simulink model "CoreXY_model_PWM_X"  (R2024b)
settings: Solver=VariableStepAuto  StartTime=0.0  StopTime=max(data.Time_ms_)/1000  RelTol=1e-3
values from neighbouring files (symbols this model uses):
  Kff = 2/PULLEY_RADIUS*(x1*s^3+x2*s^2+x3*s)    [CoreXY_analysis_func.m]    (also in feedforward_tuning.m)
undefined symbols (not defined in the file or in its folder): A, B, C, D, data, L, theta_to_xy, xy_cm_to_theta_rad
libraries: slpidlib x2
settings Model: Creator=trent  LastModifiedBy=mauro
settings OptimizationCC: ReuseModelBlockBuffer=off
settings DebuggingCC: UnconnectedInputMsg=warning  UnconnectedOutputMsg=warning  UnconnectedLineMsg=warning
settings ModelReferenceCC: EnableRefExpFcnMdlSchedulingChecks=on
settings RTWCC: GPUComputeCapability=3.5  DLArmComputeVersion=19.05

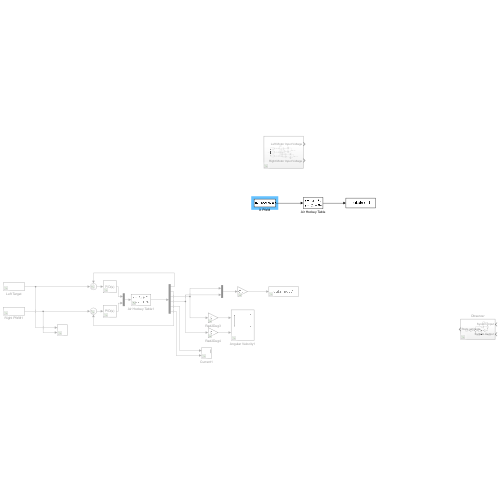
[thumbnail: Simulink's stored preview of the top-level diagram]
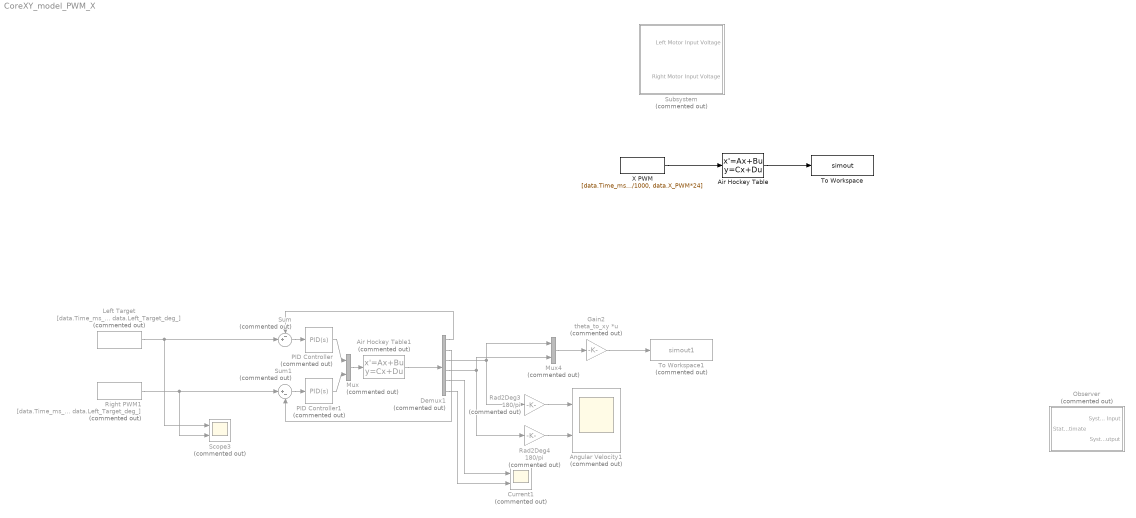
== system CoreXY_model_PWM_X ==
  Air Hockey Table : StateSpace  A=A  B=B  C=C  D=D  InitialCondition=[data.X_Accel_m_s2_(1)/C(1,3);data.X_Velocity_m_s_(1)/C(1,3);data.x(1)/C(1,3)]
  Air Hockey Table1 : StateSpace  Commented=on  A=A  B=B  C=[C; zeros(4,2) eye(4)]  D=[D; zeros(4,2)]  InitialCondition=[0;0;0;0;0;0];
  Angular Velocity1 : Scope  Commented=on  NumInputPorts=2
  Current1 : Scope  Commented=on  NumInputPorts=2
  Demux1 : Demux  Commented=on  Outputs=6
  Gain2 : Gain  Commented=on  Gain=theta_to_xy  Multiplication=Matrix(K*u)
  Left Target : FromWorkspace  Commented=on  VariableName=[data.Time_ms_/1000, data.Left_Target_deg_]
  Mux : Mux  Commented=on  Inputs=2
  Mux4 : Mux  Commented=on  Inputs=2
  Observer : Subsystem  Commented=on
  PID Controller : slpidlib/PID Controller  Commented=on  Controller=PID  Form=Parallel  TimeDomain=Continuous-time  UseExternalTs=off  SampleTime=-1  IntegratorMethod=Forward Euler  FilterMethod=Forward Euler  ControllerParametersSource=internal  P=1  I=1  UseKiTs=off  D=0  UseExternalDerivativeSource=off  N=100  UseFilter=on  TunerSelectOption=Transfer Function Based (PID Tuner App)  InitialConditionSource=internal  InitialConditionForIntegrator=0  InitialConditionForFilter=0  DifferentiatorICPrevScaledInput=0  ExternalReset=none  TrackingMode=off  Kt=1  LimitOutput=off  SatLimitsSource=internal  UpperSaturationLimit=inf  LowerSaturationLimit=-inf  LinearizeAsGain=on  AntiWindupMode=none  Kb=1  LimitIntegrator=off  UpperIntegratorSaturationLimit=inf  LowerIntegratorSaturationLimit=-inf  POutMin=[]  POutMax=[]  IOutMin=[]  IOutMax=[]  DOutMin=[]  DOutMax=[]  NOutMin=[]  NOutMax=[]  SumOutMin=[]  SumOutMax=[]  SaturationOutMin=[]  SaturationOutMax=[]  PParamMin=[]  PParamMax=[]  IParamMin=[]  IParamMax=[]  DParamMin=[]  DParamMax=[]  NParamMin=[]  NParamMax=[]  KbParamMin=[]  KbParamMax=[]  KtParamMin=[]  KtParamMax=[]  KbOutMin=[]  KbOutMax=[]  KtOutMin=[]  KtOutMax=[]  IntegratorOutMin=[]  IntegratorOutMax=[]  FilterOutMin=[]  FilterOutMax=[]  SumI1OutMin=[]  SumI1OutMax=[]  SumI2OutMin=[]  SumI2OutMax=[]  SumI3OutMin=[]  SumI3OutMax=[]  SumI4OutMin=[]  SumI4OutMax=[]  SumDOutMin=[]  SumDOutMax=[]  DifferentiatorOutMin=[]  DifferentiatorOutMax=[]  FilterDiffOutCoefMin=[]  FilterDiffOutCoefMax=[]  ReciprocalOutMin=[]  ReciprocalOutMax=[]  SumDenOutMin=[]  SumDenOutMax=[]  SumNumOutMin=[]  SumNumOutMax=[]  DivideOutMin=[]  DivideOutMax=[]  UdiffTsProdOutMin=[]  UdiffTsProdOutMax=[]  NTsProdOutMin=[]  NTsProdOutMax=[]  UintegralTsProdOutMin=[]  UintegralTsProdOutMax=[]  UngainTsProdOutMin=[]  UngainTsProdOutMax=[]  ClampingZeroOutDataTypeStr=Inherit: Inherit via back propagation  ClampingZeroOutMin=[]  ClampingZeroOutMax=[]  FilterDenConstantOutDataTypeStr=Inherit: Inherit via back propagation  FilterDenConstantOutMin=[]  FilterDenConstantOutMax=[]  PCopyOutDataTypeStr=Inherit: Inherit via back propagation  PCopyOutMin=[]  PCopyOutMax=[]  NCopyOutDataTypeStr=Inherit: Inherit via back propagation  NCopyOutMin=[]  NCopyOutMax=[]  IntegratorContinuousStateAttributes=''  IntegratorStateMustResolveToSignalObject=off  IntegratorRTWStateStorageClass=Auto  FilterContinuousStateAttributes=''  FilterStateMustResolveToSignalObject=off  FilterRTWStateStorageClass=Auto  ParallelPVariant=InternalParameters  IdealPVariant=Disabled  IVariant=InternalParameters  DVariant=InternalParameters  IntegratorVariant=Continuous  SatVariant=Disabled  AWVariant=Passthrough  PCopyVariant=Disabled  TRVariant=Disabled  FdbkBlocksVariant=Forward  IdealPFdbkVariant=Disabled  SatFdbkVariant=Disabled  DerivativeFilterVariant=ContFilter  NVariant=InternalParameters  NCopyVariant=Disabled  FilterICVariant=InternalICsFilter  IntegratorICVariant=InternalICs  ExternalResetVariant=Disabled  TRSumVariant=Passthrough  SumFdbkVariant=Disabled  SumVariant=Sum_PID  TsampFilterVariant=InternalTs  TsampNgainVariant=Passthrough  TsampIntegralVariant=Disabled_SignalSpec  ExternalSaturationOutDataTypeStr=Inherit: Same as second input  DerivativeSourceVariant=ErrorSignal  PreIntVariant=InternalPreInt
  PID Controller1 : slpidlib/PID Controller  Commented=on  Controller=PID  Form=Parallel  TimeDomain=Continuous-time  UseExternalTs=off  SampleTime=-1  IntegratorMethod=Forward Euler  FilterMethod=Forward Euler  ControllerParametersSource=internal  P=1  I=1  UseKiTs=off  D=0  UseExternalDerivativeSource=off  N=100  UseFilter=on  TunerSelectOption=Transfer Function Based (PID Tuner App)  InitialConditionSource=internal  InitialConditionForIntegrator=0  InitialConditionForFilter=0  DifferentiatorICPrevScaledInput=0  ExternalReset=none  TrackingMode=off  Kt=1  LimitOutput=off  SatLimitsSource=internal  UpperSaturationLimit=inf  LowerSaturationLimit=-inf  LinearizeAsGain=on  AntiWindupMode=none  Kb=1  LimitIntegrator=off  UpperIntegratorSaturationLimit=inf  LowerIntegratorSaturationLimit=-inf  POutMin=[]  POutMax=[]  IOutMin=[]  IOutMax=[]  DOutMin=[]  DOutMax=[]  NOutMin=[]  NOutMax=[]  SumOutMin=[]  SumOutMax=[]  SaturationOutMin=[]  SaturationOutMax=[]  PParamMin=[]  PParamMax=[]  IParamMin=[]  IParamMax=[]  DParamMin=[]  DParamMax=[]  NParamMin=[]  NParamMax=[]  KbParamMin=[]  KbParamMax=[]  KtParamMin=[]  KtParamMax=[]  KbOutMin=[]  KbOutMax=[]  KtOutMin=[]  KtOutMax=[]  IntegratorOutMin=[]  IntegratorOutMax=[]  FilterOutMin=[]  FilterOutMax=[]  SumI1OutMin=[]  SumI1OutMax=[]  SumI2OutMin=[]  SumI2OutMax=[]  SumI3OutMin=[]  SumI3OutMax=[]  SumI4OutMin=[]  SumI4OutMax=[]  SumDOutMin=[]  SumDOutMax=[]  DifferentiatorOutMin=[]  DifferentiatorOutMax=[]  FilterDiffOutCoefMin=[]  FilterDiffOutCoefMax=[]  ReciprocalOutMin=[]  ReciprocalOutMax=[]  SumDenOutMin=[]  SumDenOutMax=[]  SumNumOutMin=[]  SumNumOutMax=[]  DivideOutMin=[]  DivideOutMax=[]  UdiffTsProdOutMin=[]  UdiffTsProdOutMax=[]  NTsProdOutMin=[]  NTsProdOutMax=[]  UintegralTsProdOutMin=[]  UintegralTsProdOutMax=[]  UngainTsProdOutMin=[]  UngainTsProdOutMax=[]  ClampingZeroOutDataTypeStr=Inherit: Inherit via back propagation  ClampingZeroOutMin=[]  ClampingZeroOutMax=[]  FilterDenConstantOutDataTypeStr=Inherit: Inherit via back propagation  FilterDenConstantOutMin=[]  FilterDenConstantOutMax=[]  PCopyOutDataTypeStr=Inherit: Inherit via back propagation  PCopyOutMin=[]  PCopyOutMax=[]  NCopyOutDataTypeStr=Inherit: Inherit via back propagation  NCopyOutMin=[]  NCopyOutMax=[]  IntegratorContinuousStateAttributes=''  IntegratorStateMustResolveToSignalObject=off  IntegratorRTWStateStorageClass=Auto  FilterContinuousStateAttributes=''  FilterStateMustResolveToSignalObject=off  FilterRTWStateStorageClass=Auto  ParallelPVariant=InternalParameters  IdealPVariant=Disabled  IVariant=InternalParameters  DVariant=InternalParameters  IntegratorVariant=Continuous  SatVariant=Disabled  AWVariant=Passthrough  PCopyVariant=Disabled  TRVariant=Disabled  FdbkBlocksVariant=Forward  IdealPFdbkVariant=Disabled  SatFdbkVariant=Disabled  DerivativeFilterVariant=ContFilter  NVariant=InternalParameters  NCopyVariant=Disabled  FilterICVariant=InternalICsFilter  IntegratorICVariant=InternalICs  ExternalResetVariant=Disabled  TRSumVariant=Passthrough  SumFdbkVariant=Disabled  SumVariant=Sum_PID  TsampFilterVariant=InternalTs  TsampNgainVariant=Passthrough  TsampIntegralVariant=Disabled_SignalSpec  ExternalSaturationOutDataTypeStr=Inherit: Same as second input  DerivativeSourceVariant=ErrorSignal  PreIntVariant=InternalPreInt
  Rad2Deg3 : Gain  Commented=on  Gain=180/pi
  Rad2Deg4 : Gain  Commented=on  Gain=180/pi
  Right PWM1 : FromWorkspace  Commented=on  VariableName=[data.Time_ms_/1000, data.Left_Target_deg_]
  Scope3 : Scope  Commented=on  NumInputPorts=2
  Subsystem : Subsystem  Commented=on
  Sum : Sum  Commented=on  Inputs=-+|
  Sum1 : Sum  Commented=on  Inputs=|+-
  To Workspace : ToWorkspace  VariableName=simout  SaveFormat=Timeseries  SampleTime=-1
  To Workspace1 : ToWorkspace  Commented=on  VariableName=simout1  SaveFormat=Timeseries  SampleTime=-1
  X PWM : FromWorkspace  VariableName=[data.Time_ms_/1000, data.X_PWM*24]
  wires:
  Air Hockey Table/1 -> To Workspace/1
  Demux1/3 -> Mux4/1, Rad2Deg3/1
  Gain2/1 -> To Workspace1/1
  Mux4/1 -> Gain2/1
  Rad2Deg3/1 -> Angular Velocity1/1
  Right PWM1/1 -> Scope3/2, Sum1/1
  Demux1/4 -> Rad2Deg4/1, Mux4/2
  Demux1/6 -> Current1/2
  Demux1/5 -> Current1/1
  Left Target/1 -> Scope3/1, Sum/2
  Rad2Deg4/1 -> Angular Velocity1/2
  Mux/1 -> Air Hockey Table1/1
  PID Controller1/1 -> Mux/2
  PID Controller/1 -> Mux/1
  Air Hockey Table1/1 -> Demux1/1
  Sum/1 -> PID Controller/1
  Demux1/1 -> Sum/1
  Demux1/2 -> Sum1/2
  Sum1/1 -> PID Controller1/1
  X PWM/1 -> Air Hockey Table/1

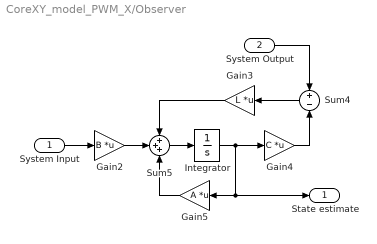
== system CoreXY_model_PWM_X/Observer ==
  System Input : Inport
  System Output : Inport  Port=2
  Gain2 : Gain  Gain=B  Multiplication=Matrix(K*u)
  Gain3 : Gain  Gain=L  Multiplication=Matrix(K*u)
  Gain4 : Gain  Gain=C  Multiplication=Matrix(K*u)
  Gain5 : Gain  Gain=A  Multiplication=Matrix(K*u)
  Integrator : Integrator
  Sum4 : Sum  Inputs=+|-
  Sum5 : Sum  Inputs=+++
  State estimate : Outport
  wires:
  System Input/1 -> Gain2/1
  Integrator/1 -> State estimate/1, Gain5/1, Gain4/1
  Gain3/1 -> Sum5/1
  Gain2/1 -> Sum5/2
  Gain5/1 -> Sum5/3
  Sum5/1 -> Integrator/1
  Sum4/1 -> Gain3/1
  Gain4/1 -> Sum4/2
  System Output/1 -> Sum4/1

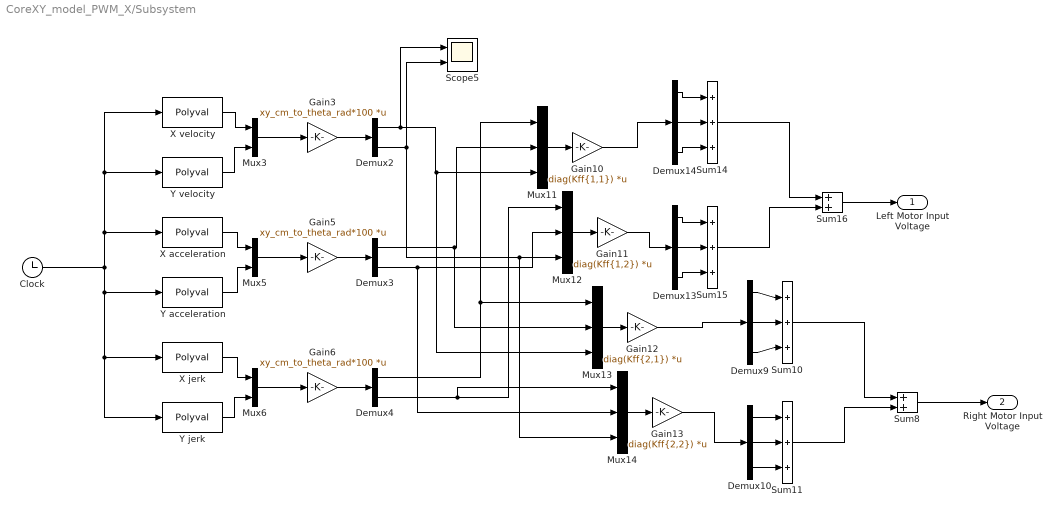
== system CoreXY_model_PWM_X/Subsystem ==
  Clock : Clock
  Demux{9..10,13..14} (4 alike) : Demux  Outputs=3
  Demux2 : Demux  Outputs=2
  Demux3 : Demux  Outputs=2
  Demux4 : Demux  Outputs=2
  Gain10 : Gain  Gain=diag(Kff{1,1})  Multiplication=Matrix(K*u)
  Gain11 : Gain  Gain=diag(Kff{1,2})  Multiplication=Matrix(K*u)
  Gain12 : Gain  Gain=diag(Kff{2,1})  Multiplication=Matrix(K*u)
  Gain13 : Gain  Gain=diag(Kff{2,2})  Multiplication=Matrix(K*u)
  Gain3 : Gain  Gain=xy_cm_to_theta_rad*100  Multiplication=Matrix(K*u)
  Gain5 : Gain  Gain=xy_cm_to_theta_rad*100  Multiplication=Matrix(K*u)
  Gain6 : Gain  Gain=xy_cm_to_theta_rad*100  Multiplication=Matrix(K*u)
  Mux{11..14} (4 alike) : Mux  Inputs=3
  Mux3 : Mux  Inputs=2
  Mux5 : Mux  Inputs=2
  Mux6 : Mux  Inputs=2
  Scope5 : Scope  NumInputPorts=2
  Sum{10..11,14..15} (4 alike) : Sum  Inputs=+++
  Sum16 : Sum
  Sum8 : Sum
  X acceleration : Polyval  Coefs=[-795.16*5*4, 867.02*4*3, -336.04*3*2, 48.83*2*1]
  X jerk : Polyval  Coefs=[-795.16*5*4*3, 867.02*4*3*2, -336.04*3*2*1]
  X velocity : Polyval  Coefs=[-795.16*5, 867.02*4, -336.04*3, 48.83*2, 0]
  Y acceleration : Polyval  Coefs=[736.08*5*4, -772.37*4*3, 275.79*3*2, -29.77*2*1]
  Y jerk : Polyval  Coefs=[736.08*5*4*3, -772.37*4*3*2, 275.79*3*2*1]
  Y velocity : Polyval  Coefs=[736.08*5, -772.37*4, 275.79*3, -29.77*2, 0]
  Left Motor Input Voltage : Outport
  Right Motor Input Voltage : Outport  Port=2
  wires:
  Clock/1 -> Y jerk/1, X jerk/1, Y acceleration/1, X acceleration/1, X velocity/1, Y velocity/1
  Mux3/1 -> Gain3/1
  Gain13/1 -> Demux10/1
  X velocity/1 -> Mux3/1
  Sum8/1 -> Right Motor Input Voltage/1
  Demux10/3 -> Sum11/3
  Y jerk/1 -> Mux6/2
  Demux9/3 -> Sum10/3
  Demux3/2 -> Mux14/2, Mux12/2
  Y acceleration/1 -> Mux5/2
  Demux10/2 -> Sum11/2
  Y velocity/1 -> Mux3/2
  Demux13/2 -> Sum15/2
  Demux4/1 -> Mux13/1, Mux11/1
  Demux9/1 -> Sum10/1
  Demux10/1 -> Sum11/1
  Demux2/2 -> Mux14/3, Mux12/3, Scope5/2
  X acceleration/1 -> Mux5/1
  Gain10/1 -> Demux14/1
  Demux4/2 -> Mux14/1, Mux12/1
  Mux6/1 -> Gain6/1
  X jerk/1 -> Mux6/1
  Sum15/1 -> Sum16/2
  Sum11/1 -> Sum8/2
  Gain6/1 -> Demux4/1
  Demux13/3 -> Sum15/3
  Mux13/1 -> Gain12/1
  Demux14/1 -> Sum14/1
  Demux2/1 -> Scope5/1, Mux13/3, Mux11/3
  Sum16/1 -> Left Motor Input Voltage/1
  Gain5/1 -> Demux3/1
  Gain12/1 -> Demux9/1
  Demux9/2 -> Sum10/2
  Sum10/1 -> Sum8/1
  Mux5/1 -> Gain5/1
  Demux14/3 -> Sum14/3
  Gain3/1 -> Demux2/1
  Mux14/1 -> Gain13/1
  Gain11/1 -> Demux13/1
  Demux3/1 -> Mux13/2, Mux11/2
  Mux11/1 -> Gain10/1
  Sum14/1 -> Sum16/1
  Demux14/2 -> Sum14/2
  Demux13/1 -> Sum15/1
  Mux12/1 -> Gain11/1
